simulink model "and_switch_dashboard"  (R2018b)
settings: Solver=VariableStepAuto  StartTime=0.0  StopTime=40  RelTol=1e-3
settings Model: EnablePacing=on  Creator=kjartan  LastModifiedBy=kjartan

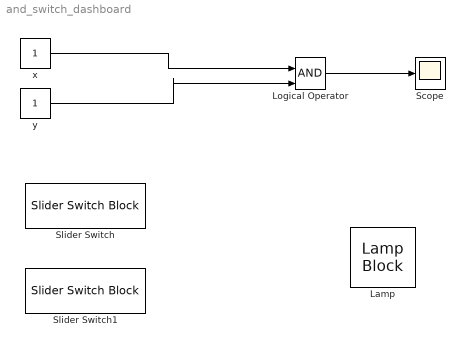
== system and_switch_dashboard ==
  Lamp : LampBlock  WebBlockId=4
  Logical Operator : Logic  IconShape=distinctive  AllPortsSameDT=off  OutDataTypeStr=boolean
  Scope : Scope
  Slider Switch : SliderSwitchBlock  WebBlockId=2
      settings: Values={{'Off', 'On'}, [0 1]}
  Slider Switch1 : SliderSwitchBlock  WebBlockId=14
      settings: Values={{'Off', 'On'}, [0 1]}
  x : Constant
  y : Constant
  wires:
  Logical Operator/1 -> Scope/1
  x/1 -> Logical Operator/1
  y/1 -> Logical Operator/2
